simulink model "Circuito_RLC"  (R2021b)
settings: Solver=VariableStepAuto  StartTime=0.0  StopTime=10.0  RelTol=1e-3
values from neighbouring files (symbols this model uses):
  C = 1    [RLC_PARAMETROS.m]
  L = 1    [RLC_PARAMETROS.m]
  R = 2    [RLC_PARAMETROS.m]
  v = 5    [RLC_PARAMETROS.m]
settings Model: Creator=mluser  LastModifiedBy=mluser

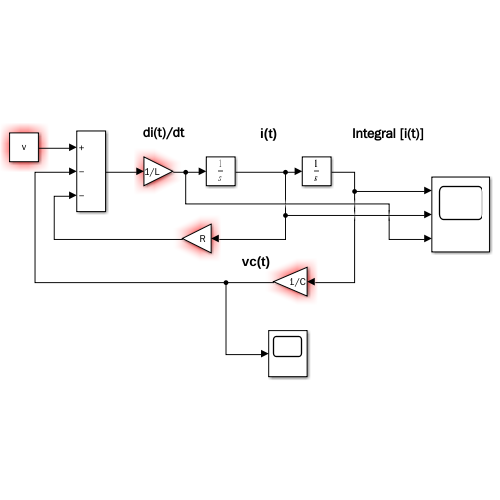
[thumbnail: Simulink's stored preview of the top-level diagram]
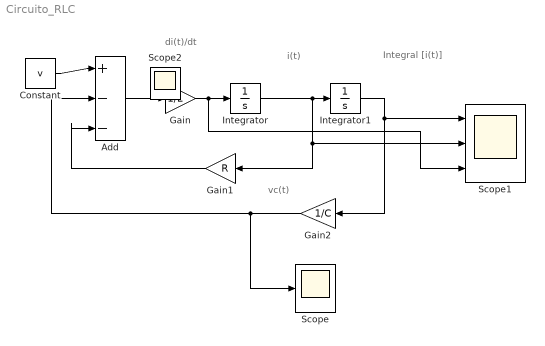
== system Circuito_RLC ==
  note: Integral [i(t)]
  note: i(t)
  note: di(t)/dt
  note: vc(t)
  Add : Sum  Inputs=+--
  Constant : Constant  Value=v
  Gain : Gain  Gain=1/L
  Gain1 : Gain  Gain=R
  Gain2 : Gain  Gain=1/C
  Integrator : Integrator
  Integrator1 : Integrator
  Scope : Scope
  Scope1 : Scope  NumInputPorts=3
  Scope2 : Scope
  wires:
  Integrator/1 -> Scope1/2, Gain1/1, Integrator1/1
  Constant/1 -> Add/1
  Gain1/1 -> Add/3
  Integrator1/1 -> Gain2/1, Scope1/1
  Gain2/1 -> Scope/1, Add/2
  Gain/1 -> Scope1/3, Integrator/1
  Add/1 -> Gain/1
